simulink model "PCM"  (R2016b)
settings: Solver=VariableStepAuto  StartTime=0.0  StopTime=10.0  RelTol=1e-3
libraries: commsrccod2 x1, commutil2 x1
settings Model: Creator=white  LastModifiedBy=white

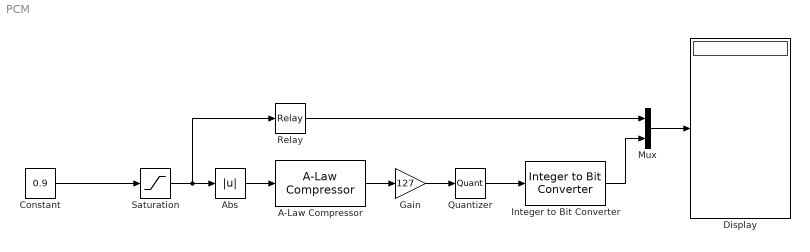
== system PCM ==
  A-Law Compressor : commsrccod2/A-Law Compressor  A=87.6  V=1
  Abs : Abs
  Constant : Constant  Value=0.9
  Display : Display
      settings: Format=binary (Stored Integer)  Decimation=8
  Gain : Gain  Gain=127
  Integer to Bit Converter : commutil2/Integer to Bit Converter  nbits=7  signedInputValues=Unsigned  bitOrder=MSB first  outDtype=Inherit via internal rule
  Mux : Mux  Inputs=2
  Quantizer : Quantizer  QuantizationInterval=1
  Relay : Relay  OnSwitchValue=0  OffSwitchValue=0  OnOutputValue=0  OffOutputValue=1
  Saturation : Saturate  UpperLimit=1  LowerLimit=-1
  wires:
  Saturation/1 -> Relay/1, Abs/1
  Abs/1 -> A-Law Compressor/1
  Integer to Bit Converter/1 -> Mux/2
  Relay/1 -> Mux/1
  A-Law Compressor/1 -> Gain/1
  Gain/1 -> Quantizer/1
  Quantizer/1 -> Integer to Bit Converter/1
  Constant/1 -> Saturation/1
  Mux/1 -> Display/1
